simulink model "gps_simulate_1sat_demo"  (Simulink 7.3)
settings: Solver=ode45  StartTime=0.0  StopTime=86400  RelTol=1e-3
undefined symbols (not defined in the file): WGS
libraries: rapidstm32_gps_lib x5
settings Model: Creator=Compaq  LastModifiedBy=Compaq

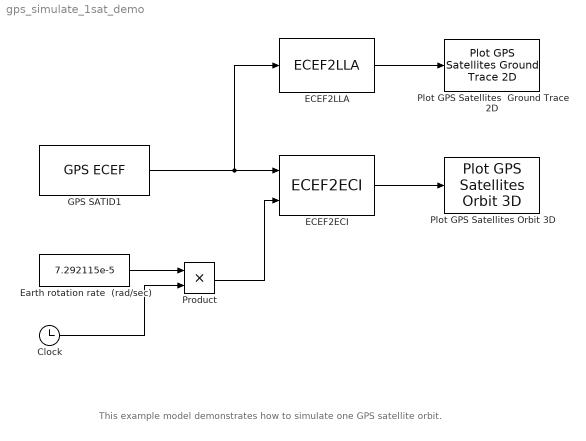
== system gps_simulate_1sat_demo ==
  note: This example model demonstrates how to simulate one GPS satellite orbit.
  Clock : Clock
      settings: Decimation=10
  ECEF2ECI : rapidstm32_gps_lib/ECEF2ECI
  ECEF2LLA : rapidstm32_gps_lib/ECEF2LLA  latlong_format=Degrees  altitude_format=Meters  refellipsoid=WGS-84  re=6378137  epsilon=0.081819190842622
  Earth rotation rate  (rad/sec) : Constant  Value=7.292115e-5  OutDataType=fixdt(1, 16)  OutScaling=2^0
  GPS SATID1 : rapidstm32_gps_lib/GPS ECEF  satid=19  t0=0  sampletime=600
  Plot GPS Satellites  Ground Trace 2D : rapidstm32_gps_lib/Plot GPS Satellites Ground Trace 2D  satid_all=off  satid1=off  satid2=off  satid3=off  satid4=off  satid5=off  satid6=off  satid7=off  satid8=off  satid9=off  satid10=off  satid11=off  satid12=off  satid13=off  satid14=off  satid15=off  satid16=off  satid17=off  satid18=off  satid19=on  satid20=off  satid21=off  satid22=off  satid23=off  satid24=off  visibility_vec=No
  Plot GPS Satellites Orbit 3D : rapidstm32_gps_lib/Plot GPS Satellites Orbit 3D  satid_all=off  satid1=off  satid2=off  satid3=off  satid4=off  satid5=off  satid6=off  satid7=off  satid8=off  satid9=off  satid10=off  satid11=off  satid12=off  satid13=off  satid14=off  satid15=off  satid16=off  satid17=off  satid18=off  satid19=on  satid20=off  satid21=off  satid22=off  satid23=off  satid24=off  visibility_vec=No
  Product : Product  OutDataType=fixdt(1, 16)  OutScaling=2^0  RndMeth=Zero
  wires:
  Earth rotation rate  (rad/sec)/1 -> Product/1
  Clock/1 -> Product/2
  GPS SATID1/1 -> ECEF2ECI/1, ECEF2LLA/1
  ECEF2ECI/1 -> Plot GPS Satellites Orbit 3D/1
  Product/1 -> ECEF2ECI/2
  ECEF2LLA/1 -> Plot GPS Satellites  Ground Trace 2D/1
